simulink model "ShiftLogic"  (R2023b)
settings: Solver=FixedStepDiscrete  StartTime=0.0  StopTime=10.0  FixedStep=0.04  RelTol=1e-3
model workspace (MAT data in the model file):
  DOWN_TABLE = [0  31.66  54.01  79.62; 0  31.66  54.01  79.62; 0  31.54  53.79  79.36; 0  31.45  53.62  79.18; 0  31.36  53.45  78.98; 0  31.34  53.43  78.96]
  DOWN_TH_BP = [0; 25; 35; 50; 90; 100]
  UP_TABLE = [36.66  59.01  84.62; 36.66  59.01  84.62; 36.54  58.79  84.36; 36.45  58.62  84.18; 36.36  58.45  83.98; 36.34  58.43  83.96]
  UP_TH_BP = [0; 25; 35; 50; 90; 100]
settings Model: Creator=muzing  LastModifiedBy=muzing

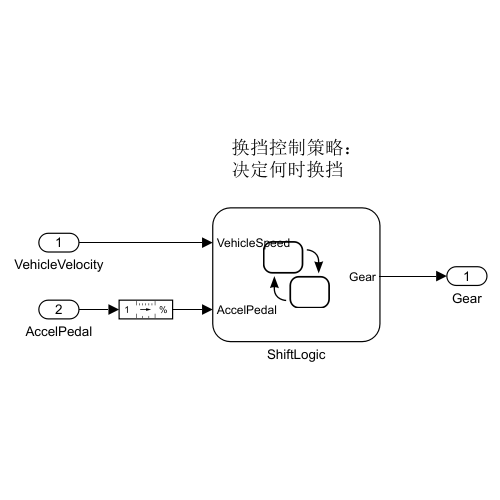
[thumbnail: Simulink's stored preview of the top-level diagram]
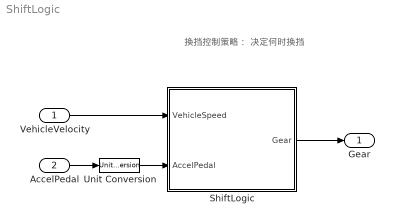
== system ShiftLogic ==
  note: 换挡控制策略：
      | 决定何时换挡
  VehicleVelocity : Inport  Unit=km/h
  AccelPedal : Inport  Port=2  Unit=1
  ShiftLogic : Stateflow chart  TreatAsAtomicUnit=on
      settings: PortSchema="{\"entries\":[{\"content\":{\"sides\":[{\"content\":{\"connectorIds\":[\"In2\",\"In1\"]},\"type\":\"ConnectorPlacement.EquallySpacedRectSide\",\"uuid\":\"8d1a78b0-e131-4d32-aab6-f273cb65ea30\"},{\"content\":{\"connectorIds\":[\"Out1\"],\"side\":\"RIGHT\"},\"type\":\"ConnectorPlacement.EquallySpacedRectSide\",\"uuid\":\"bf2d0fc6-ae88-4278-a7fe-de26814c6b0c\"},{\"content\":{\"side\":\"TOP\"},\"type\":\"ConnectorPlacement.EquallySpacedRectSide\",\"uuid\":\"7546cb3c-129a-4268-9a81-c22f80bf2078\"}]},\"type\":\"ConnectorPlacement.EquallySpacedConnector\",\"uuid\":\"205ae68e-ffaa-4987-8afa-8e6f731975e5\"}],\"packageUris\":[\"http://schema.mathworks.com/mf0/Connector/R2020b\"],\"version\":\"1.0\"}"
  Unit Conversion : UnitConversion
  Gear : Outport
  wires:
  AccelPedal/1 -> Unit Conversion/1
  ShiftLogic/1(Gear) -> Gear/1
  VehicleVelocity/1 -> ShiftLogic/2(VehicleSpeed)
  Unit Conversion/1 -> ShiftLogic/1(AccelPedal)

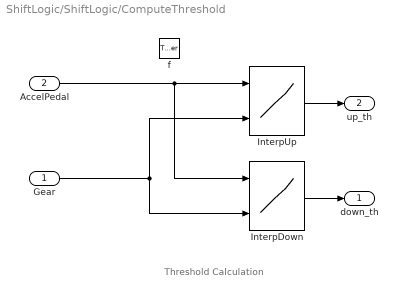
== system ShiftLogic/ShiftLogic/ComputeThreshold ==
  note: Threshold Calculation
  Gear : Inport
  AccelPedal : Inport  Port=2
  f : TriggerPort  TriggerType=function-call  VariantControl=(inherit)
      settings: CopyFcn=Stateflow.SLINSF.SimulinkMan.removeBlockPreDeleteFcn  PreDeleteFcn=Stateflow.SLINSF.SimulinkMan.unsafePredeleteFcn
  InterpDown : Lookup_n-D  BreakpointsForDimension1=DOWN_TH_BP  BreakpointsForDimension2=[1:4]  Table=DOWN_TABLE  OutDataTypeStr=double  InputSameDT=off  LockScale=on
      settings: InputPortMap=u0,u1
  InterpUp : Lookup_n-D  BreakpointsForDimension1=UP_TH_BP  BreakpointsForDimension2=[1:3]  Table=UP_TABLE  OutDataTypeStr=double  InputSameDT=off  LockScale=on
      settings: InputPortMap=u0,u1
  down_th : Outport  InitialOutput=0  VectorParamsAs1DForOutWhenUnconnected=off
  up_th : Outport  Port=2  InitialOutput=0  VectorParamsAs1DForOutWhenUnconnected=off
  wires:
  InterpUp/1 -> up_th/1
  InterpDown/1 -> down_th/1
  Gear/1 -> InterpDown/2, InterpUp/2
  AccelPedal/1 -> InterpDown/1, InterpUp/1

== stateflow chart ShiftLogic/ShiftLogic ==
  settings: updateMethod=DISCRETE  sampleTime=0.04
  state gear_state [parallel]
    settings: executionOrder=1
    state first
      entry:
      Gear = 1;
    state second
      entry:
      Gear = 2;
    state third
      entry:
      Gear = 3;
    state fourth
      entry:
      Gear = 4;
    (default) -> first
    second -> third [order 1] : UP
    first -> second : UP
    third -> fourth [order 1] : UP
    third -> second [order 2] : DOWN
    second -> first [order 2] : DOWN
    fourth -> third : DOWN
  state selection_state [parallel]
    during:
    [down_th, up_th] = ComputeThreshold(Gear,AccelPedal);
    settings: executionOrder=2
    state steady_state
    state upshifting
    state downshifting
    (default) -> steady_state
    steady_state -> upshifting [order 1] : [VehicleSpeed > up_th]
    steady_state -> downshifting [order 2] : [VehicleSpeed < down_th]
    downshifting -> steady_state [order 2] : [VehicleSpeed > down_th]
    downshifting -> steady_state [order 1] : after(2,tick)
        | [VehicleSpeed <= down_th]
        | {gear_state.DOWN}
    upshifting -> steady_state [order 1] : after(2,tick)
        | [VehicleSpeed >= up_th]
        | {gear_state.UP}
    upshifting -> steady_state [order 2] : [VehicleSpeed < up_th]
  state [down_th,up_th] = ComputeThreshold(Gear,AccelPedal) [function]
  data: Gear function_input; AccelPedal function_input; down_th function_output; up_th function_output; AccelPedal input double; VehicleSpeed input double; Gear output double [1..4]; down_th local double; up_th local double
  events: DOWN local EITHER_EDGE_EVENT; UP local EITHER_EDGE_EVENT
